simulink model "tc_Riccati_solve"  (Simulink 8.9)
settings: Solver=ode3  StartTime=0.0  StopTime=T  FixedStep=0.01  RelTol=1e-3  EnableMultiTasking=on
values from neighbouring files (symbols this model uses):
  A = [0 1; 0 0]    [Week6_prob2.m]
  B = [0;1]    [Week6_prob2.m]
  Q = [2 1; 1 4]    [Week6_prob2.m]
  R = 1/2    (= 0.5)    [Week6_prob2.m]
  Z = [1 0; 0 2]    [Week6_prob2.m]
settings Model: Creator=Thomas Chmielewski  LastModifiedBy=DR_C
settings OptimizationCC: ExpressionDepthLimit=2147483647
settings DebuggingCC: SolverPrmCheckMsg=warning  AllowSymbolicDim=off
settings ConfigComp: CovSFcnEnable=off

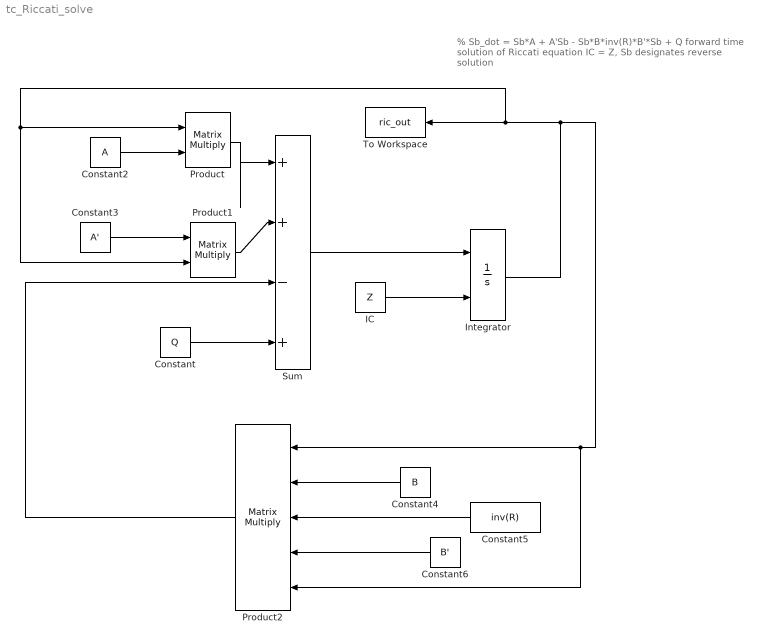
== system tc_Riccati_solve ==
  note: % Sb_dot = Sb*A + A'Sb - Sb*B*inv(R)*B'*Sb + Q
      | forward time solution of Riccati equation
      | IC = Z, Sb designates reverse solution
  Constant : Constant  Value=Q  VectorParams1D=off
  Constant2 : Constant  Value=A  VectorParams1D=off
  Constant3 : Constant  Value=A'  VectorParams1D=off
  Constant4 : Constant  Value=B  VectorParams1D=off
  Constant5 : Constant  Value=inv(R)  VectorParams1D=off
  Constant6 : Constant  Value=B'  VectorParams1D=off
  IC : Constant  Value=Z  VectorParams1D=off
  Integrator : Integrator  InitialConditionSource=external
  Product : Product  Multiplication=Matrix(*)  RndMeth=Zero
  Product1 : Product  Multiplication=Matrix(*)  RndMeth=Zero
  Product2 : Product  Inputs=5  Multiplication=Matrix(*)  RndMeth=Zero
  Sum : Sum  Inputs=|++-+
  To Workspace : ToWorkspace  VariableName=ric_out  SaveFormat=Structure With Time  SampleTime=-1
  wires:
  Constant/1 -> Sum/4
  IC/1 -> Integrator/2
  Product/1 -> Sum/1
  Constant2/1 -> Product/2
  Integrator/1 -> Product/1, Product1/2, To Workspace/1, Product2/1, Product2/5
  Product1/1 -> Sum/2
  Constant3/1 -> Product1/1
  Product2/1 -> Sum/3
  Constant4/1 -> Product2/2
  Constant5/1 -> Product2/3
  Constant6/1 -> Product2/4
  Sum/1 -> Integrator/1
